simulink model "verify_Storage_Type_4_CONF_mdl"  (R2016b)
settings: Solver=ode45  StartTime=0  StopTime=24*3600  MaxStep=600  RelTol=1e-3  EnableMultiTasking=on
undefined symbols (not defined in the file or in its folder): path_carnot
libraries: carnot x12, simulink x3
settings Model: Creator=drhf  LastModifiedBy=drhf
settings DataIOCC: SaveFormat=Array  SignalLoggingSaveFormat=ModelDataLogs
settings OptimizationCC: ExpressionDepthLimit=2147483647  LifeSpan=inf
settings DebuggingCC: UnderspecifiedInitializationDetection=Classic  MergeDetectMultiDrivingBlocksExec=none  SolverPrmCheckMsg=warning  FcnCallInpInsideContextMsg=warning  StateNameClashWarn=warning  SFUnexpectedBacktrackingDiag=warning  SFNoUnconditionalDefaultTransitionDiag=warning  SFExecutionAtInitializationDiag=none
settings HardwareCC: ProdBitPerPointer=32  ProdBitPerSizeT=32  ProdBitPerPtrDiffT=32  ProdLargestAtomicFloat=None  ProdIntDivRoundTo=Undefined  ProdEndianess=Unspecified  ProdWordSize=32  ProdHWDeviceType=32-bit Generic
settings ModelReferenceCC: PropagateSignalLabelsOutOfModel=off
settings GRTTargetCC: TargetLangStandard=C89/C90 (ANSI)  GeneratePreprocessorConditionals=Disable all  CombineOutputUpdateFcns=off  GRTInterface=on
settings ConfigComp: CovMetricSettings=dw  CovHtmlReporting=on  CovSaveCumulativeToWorkspaceVar=on  CovSaveSingleToWorkspaceVar=on  CovExternalEMLEnable=off

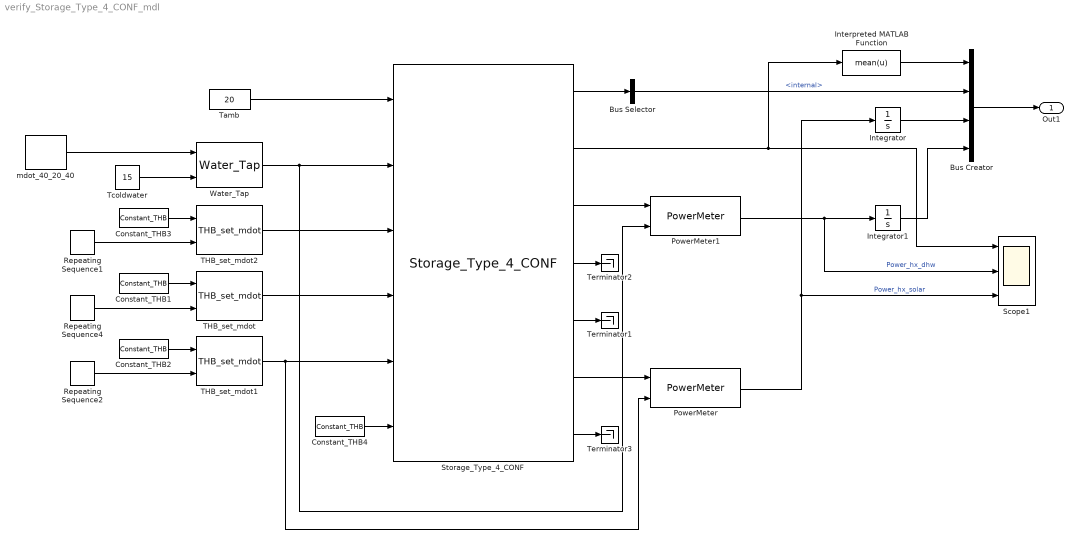
== system verify_Storage_Type_4_CONF_mdl ==
  Bus Creator : BusCreator  Inputs=4
  Bus Selector : BusSelector  OutputSignals=energy.internal
  Constant_THB1 : carnot/Source/Simple/Constant_THB  t=30  mdot=100/3600  p=1e5  mID=Full Pressure Drop with Static Height  fluid=Water  mix=0  mix2=0  mix3=0  dia=0.02  hgt=0
  Constant_THB2 : carnot/Source/Simple/Constant_THB  t=40  mdot=100/3600  p=1e5  mID=Full Pressure Drop with Static Height  fluid=Water  mix=0  mix2=0  mix3=0  dia=0.02  hgt=0
  Constant_THB3 : carnot/Source/Simple/Constant_THB  t=60  mdot=0  p=1e5  mID=Full Pressure Drop with Static Height  fluid=Water  mix=0  mix2=0  mix3=0  dia=0.02  hgt=0
  Constant_THB4 : carnot/Source/Simple/Constant_THB  t=20  mdot=0  p=1e5  mID=Full Pressure Drop with Static Height  fluid=Water  mix=0  mix2=0  mix3=0  dia=0.02  hgt=0
  Integrator : Integrator
  Integrator1 : Integrator
  Interpreted MATLAB Function : MATLABFcn  MATLABFcn=mean(u)
  PowerMeter : carnot/Control/PowerMeter
  PowerMeter1 : carnot/Control/PowerMeter
  Repeating Sequence1 : simulink/Sources/Repeating Sequence  rep_seq_t=[ 0 3600 3600+eps(3600) 7200 7200+eps(7200) 10800]  rep_seq_y=[ 0 0 0.1+0*eps(3600) 0.1 0.15+0*eps(7200) 0.15]
  Repeating Sequence2 : simulink/Sources/Repeating Sequence  rep_seq_t=[ 0 3600 3600+eps(3600) 7200 7200+eps(7200) 10800]  rep_seq_y=[ 0.12 0.12 0.11+0*eps(3600) 0.11 0.05+0*eps(7200) 0.05]
  Repeating Sequence4 : simulink/Sources/Repeating Sequence  rep_seq_t=[ 0 3600 3600+eps(3600) 7200 7200+eps(7200) 10800]  rep_seq_y=[ 0.11 0.11 0.1+0*eps(3600) 0.1 0.11+0*eps(7200) 0.11]
  Scope1 : Scope  NumInputPorts=3
  Storage_Type_4_CONF : carnot/Storage/Thermal/Storage_Type_4_CONF  t0=[10:5:55]  hgt=1.8082  stgtype=4  tini=[10 12.3684210526316 14.7368421052632 17.1052631578947 19.4736842105263 21.8421052631579 24.2105263157895 26.5789473684211 28.9473684210526 31.3157894736842 33.6842105263158 36.0526315789474 38.4210526315789 40.7894736842105 43.1578947368421 45.5263157894737 47.8947368421053 50.2631578947368 52.6315789473684 55]  mpts=[1 3 5 7 9 11 13 15 17 19]  PathName=fullfile(path_carnot('libsl'),'Storage','Thermal','Storage_Type_4_CONF','parameter_set')  FileName='StorageType4_600_L.mat'  userPath=off  userParam=off  uwall=1  ubot=1  utop=1  axcond=1  volume=0.6  dia=0.65  standing=standing cylinder  nodes=20  mpoints=10  Tsensor=[0.2 0.5 0.7]  pipe3inlet=1  pipe3outlet=0.6  pipe3dia=0.05  hx1inlet=0.4  hx1outlet=0  hx1dia=0.03  hx1uac=200  hx1uam=0.15  hx1uat=0.6  hx1dplin=20  hx1dpqua=20  pipe2inlet=0.45  pipe2outlet=0.55  pipe2dia=0.05  hx2inlet=0  hx2outlet=1  hx2dia=0.025  hx2uac=450  hx2uam=0.4  hx2uat=0.8  hx2dplin=200  hx2dpqua=200  hx3inlet=0.9  hx3outlet=1  hx3dia=0.01  hx3uac=100  hx3uam=0  hx3uat=0  hx3dplin=10  hx3dpqua=10
  THB_set_mdot : carnot/Source/Simple/THB_set_mdot
  THB_set_mdot1 : carnot/Source/Simple/THB_set_mdot
  THB_set_mdot2 : carnot/Source/Simple/THB_set_mdot
  Tamb : Constant  Value=20
  Tcoldwater : Constant  Value=15
  Terminator1 : Terminator
  Terminator2 : Terminator
  Terminator3 : Terminator
  Water_Tap : carnot/Load/Hot_Water_Tapping/Water_Tap  dia=0.02  p=2e5
  mdot_40_20_40 : carnot/Load/Hot_Water_Tapping/mdot_40_20_40  period=24*3600  rep_seq_t=[7 12 19]*3600  rep_seq_d=[0.2 0.1 0.2]*3600  rep_seq_y=[1 1 1]*200/1800
  Out1 : Outport
  wires:
  Bus Creator/1 -> Out1/1
  Tamb/1 -> Storage_Type_4_CONF/1
  Constant_THB1/1 -> THB_set_mdot/1
  THB_set_mdot/1 -> Storage_Type_4_CONF/4
  THB_set_mdot1/1 -> Storage_Type_4_CONF/5, PowerMeter/2
  Constant_THB2/1 -> THB_set_mdot1/1
  Repeating Sequence4/1 -> THB_set_mdot/2
  Repeating Sequence2/1 -> THB_set_mdot1/2
  Storage_Type_4_CONF/1 -> Bus Selector/1
  Storage_Type_4_CONF/6 -> PowerMeter/1
  PowerMeter/1 -> Scope1/3, Integrator/1  "Power_hx_solar"
  PowerMeter1/1 -> Scope1/2, Integrator1/1  "Power_hx_dhw"
  Storage_Type_4_CONF/2 -> Scope1/1, Interpreted MATLAB Function/1
  mdot_40_20_40/1 -> Water_Tap/1
  Tcoldwater/1 -> Water_Tap/2
  Bus Selector/1 -> Bus Creator/2  "<internal>"
  Storage_Type_4_CONF/4 -> Terminator2/1
  Constant_THB3/1 -> THB_set_mdot2/1
  Repeating Sequence1/1 -> THB_set_mdot2/2
  THB_set_mdot2/1 -> Storage_Type_4_CONF/3
  Integrator/1 -> Bus Creator/3
  Integrator1/1 -> Bus Creator/4
  Storage_Type_4_CONF/7 -> Terminator3/1
  Constant_THB4/1 -> Storage_Type_4_CONF/6
  Storage_Type_4_CONF/5 -> Terminator1/1
  Storage_Type_4_CONF/3 -> PowerMeter1/1
  Water_Tap/1 -> Storage_Type_4_CONF/2, PowerMeter1/2
  Interpreted MATLAB Function/1 -> Bus Creator/1
